simulink model "assignment2"  (R2020b)
settings: Solver=VariableStepAuto  StartTime=0.0  StopTime=10.0  RelTol=1e-3
undefined symbols (not defined in the file or in its folder): be, bv, Ie, Iv
settings Model: Creator=Sudhanshu  LastModifiedBy=Sudhanshu

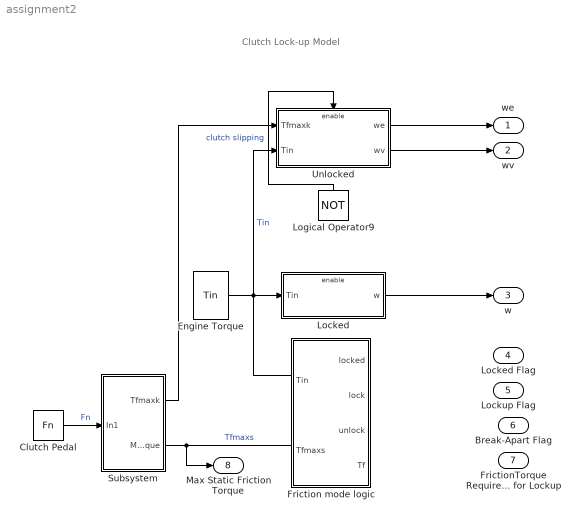
== system assignment2 ==
  note: Clutch Lock-up Model
  Clutch Pedal : FromWorkspace  VariableName=Fn  ZeroCross=off
  Engine Torque : FromWorkspace  VariableName=Tin  ZeroCross=off
  Friction mode logic : Subsystem
  Locked : Subsystem  TreatAsAtomicUnit=on
  Logical Operator9 : Logic  Operator=NOT  Inputs=1  IconShape=distinctive  OutDataTypeStr=boolean
  Subsystem : Subsystem
  Unlocked : Subsystem  TreatAsAtomicUnit=on
  we : Outport  InitialOutput=0  VectorParamsAs1DForOutWhenUnconnected=off
  wv : Outport  Port=2  InitialOutput=0  VectorParamsAs1DForOutWhenUnconnected=off
  w : Outport  Port=3  InitialOutput=0  VectorParamsAs1DForOutWhenUnconnected=off
  Locked Flag : Outport  Port=4  InitialOutput=0  VectorParamsAs1DForOutWhenUnconnected=off
  Lockup Flag : Outport  Port=5  InitialOutput=0  VectorParamsAs1DForOutWhenUnconnected=off
  Break-Apart Flag : Outport  Port=6  InitialOutput=0  VectorParamsAs1DForOutWhenUnconnected=off
  FrictionTorque Required for Lockup : Outport  Port=7  InitialOutput=0  VectorParamsAs1DForOutWhenUnconnected=off
  Max Static Friction Torque : Outport  Port=8  InitialOutput=0  VectorParamsAs1DForOutWhenUnconnected=off
  wires:
  Engine Torque/1 -> Locked/1(Tin), Unlocked/2(Tin)  "Tin"
  Unlocked/2(wv) -> wv/1
  Unlocked/1(we) -> we/1
  Logical Operator9/1 -> Unlocked/Enable  "clutch slipping"
  Locked/1(w) -> w/1
  Subsystem/1(Tfmaxk) -> Unlocked/1(Tfmaxk)
  Subsystem/2(Max Static Friction Torque) -> Max Static Friction Torque/1  "Tfmaxs"
  Clutch Pedal/1 -> Subsystem/1(In1)  "Fn"
  ? -> Locked/Enable, Logical Operator9/1, Locked Flag/1
  ? -> Lockup Flag/1
  ? -> Break-Apart Flag/1
  ? -> FrictionTorque Required for Lockup/1

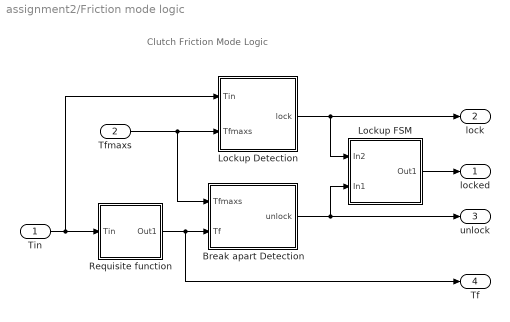
== system assignment2/Friction mode logic ==
  note: Clutch Friction Mode Logic
  Tin : Inport
  Tfmaxs : Inport  Port=2
  Break apart Detection : Subsystem
  Lockup Detection : Subsystem
  Lockup FSM : Subsystem
  Requisite function : Subsystem
  locked : Outport  InitialOutput=0  VectorParamsAs1DForOutWhenUnconnected=off
  lock : Outport  Port=2  InitialOutput=0  VectorParamsAs1DForOutWhenUnconnected=off
  unlock : Outport  Port=3  InitialOutput=0  VectorParamsAs1DForOutWhenUnconnected=off
  Tf : Outport  Port=4  InitialOutput=0  VectorParamsAs1DForOutWhenUnconnected=off
  wires:
  Break apart Detection/1(unlock) -> Lockup FSM/2(In1), unlock/1
  Tfmaxs/1 -> Break apart Detection/1(Tfmaxs), Lockup Detection/2(Tfmaxs)
  Lockup FSM/1(Out1) -> locked/1
  Lockup Detection/1(lock) -> Lockup FSM/1(In2), lock/1
  Requisite function/1(Out1) -> Break apart Detection/2(Tf), Tf/1
  Tin/1 -> Lockup Detection/1(Tin), Requisite function/1(Tin)

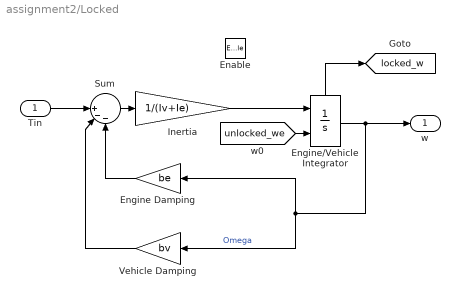
== system assignment2/Locked ==
  Tin : Inport
  Enable : EnablePort  StatesWhenEnabling=reset
  Engine Damping : Gain  Gain=be  SaturateOnIntegerOverflow=on  OutDataTypeStr=Inherit: Same as input  ParamDataTypeStr=Inherit: Same as input
  Engine/Vehicle Integrator : Integrator  InitialConditionSource=external  ShowStatePort=on
  Inertia : Gain  Gain=1/(Iv+Ie)  SaturateOnIntegerOverflow=on  OutDataTypeStr=Inherit: Same as input  ParamDataTypeStr=Inherit: Same as input
  Sum : Sum  Inputs=||+--  InputSameDT=on  SaturateOnIntegerOverflow=on  OutDataTypeStr=Inherit: Same as first input
  Vehicle Damping : Gain  Gain=bv  SaturateOnIntegerOverflow=on  OutDataTypeStr=Inherit: Same as input  ParamDataTypeStr=Inherit: Same as input
  w : Outport  InitialOutput=0  VectorParamsAs1DForOutWhenUnconnected=off
  tag scope: locked_w=global
  wires:
  Tin/1 -> Sum/1
  Engine/Vehicle Integrator/1 -> w/1, Engine Damping/1, Vehicle Damping/1  "Omega"
  Engine Damping/1 -> Sum/3
  Inertia/1 -> Engine/Vehicle Integrator/1
  Vehicle Damping/1 -> Sum/2
  Engine/Vehicle Integrator/State -> [locked_w]
  Sum/1 -> Inertia/1
  [unlocked_we] -> Engine/Vehicle Integrator/2

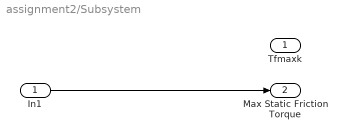
== system assignment2/Subsystem ==
  In1 : Inport
  Tfmaxk : Outport
  Max Static Friction Torque : Outport  Port=2
  wires:
  In1/1 -> Max Static Friction Torque/1

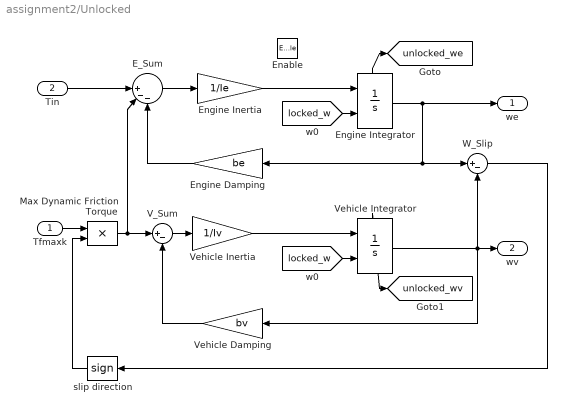
== system assignment2/Unlocked ==
  Tfmaxk : Inport
  Tin : Inport  Port=2
  Enable : EnablePort  StatesWhenEnabling=reset
  E_Sum : Sum  Inputs=||+--  InputSameDT=on  SaturateOnIntegerOverflow=on  OutDataTypeStr=Inherit: Same as first input
  Engine Damping : Gain  Gain=be  SaturateOnIntegerOverflow=on  OutDataTypeStr=Inherit: Same as input  ParamDataTypeStr=Inherit: Same as input
  Engine Inertia : Gain  Gain=1/Ie  SaturateOnIntegerOverflow=on  OutDataTypeStr=Inherit: Same as input  ParamDataTypeStr=Inherit: Same as input
  Engine Integrator : Integrator  InitialConditionSource=external  ShowStatePort=on
  Max Dynamic Friction Torque : Product  InputSameDT=on  RndMeth=Zero  SaturateOnIntegerOverflow=on  OutDataTypeStr=Inherit: Same as first input
  V_Sum : Sum  Inputs=|+-  InputSameDT=on  SaturateOnIntegerOverflow=on  OutDataTypeStr=Inherit: Same as first input
  Vehicle Damping : Gain  Gain=bv  SaturateOnIntegerOverflow=on  OutDataTypeStr=Inherit: Same as input  ParamDataTypeStr=Inherit: Same as input
  Vehicle Inertia : Gain  Gain=1/Iv  SaturateOnIntegerOverflow=on  OutDataTypeStr=Inherit: Same as input  ParamDataTypeStr=Inherit: Same as input
  Vehicle Integrator : Integrator  InitialConditionSource=external  ShowStatePort=on
  W_Slip : Sum  Inputs=|+-  InputSameDT=on  SaturateOnIntegerOverflow=on  OutDataTypeStr=Inherit: Same as first input
  slip direction : Signum
  we : Outport  InitialOutput=0  VectorParamsAs1DForOutWhenUnconnected=off
  wv : Outport  Port=2  InitialOutput=0  VectorParamsAs1DForOutWhenUnconnected=off
  tag scope: unlocked_we=global, unlocked_wv=global
  wires:
  V_Sum/1 -> Vehicle Inertia/1
  Engine Inertia/1 -> Engine Integrator/1
  [locked_w] -> Engine Integrator/2
  Engine Damping/1 -> E_Sum/3
  slip direction/1 -> Max Dynamic Friction Torque/2
  E_Sum/1 -> Engine Inertia/1
  Vehicle Integrator/State -> [unlocked_wv]
  [locked_w] -> Vehicle Integrator/2
  W_Slip/1 -> slip direction/1
  Tfmaxk/1 -> Max Dynamic Friction Torque/1
  Tin/1 -> E_Sum/1
  Vehicle Damping/1 -> V_Sum/2
  Vehicle Integrator/1 -> wv/1, W_Slip/2, Vehicle Damping/1
  Vehicle Inertia/1 -> Vehicle Integrator/1
  Engine Integrator/State -> [unlocked_we]
  Max Dynamic Friction Torque/1 -> V_Sum/1, E_Sum/2
  Engine Integrator/1 -> we/1, Engine Damping/1, W_Slip/1

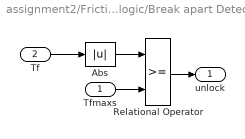
== system assignment2/Friction mode logic/Break apart Detection ==
  Tfmaxs : Inport
  Tf : Inport  Port=2
  Abs : Abs  SaturateOnIntegerOverflow=on
  Relational Operator : RelationalOperator  OutDataTypeStr=boolean  RndMeth=Nearest  InputSameDT=on
  unlock : Outport  InitialOutput=0  VectorParamsAs1DForOutWhenUnconnected=off
  wires:
  Abs/1 -> Relational Operator/1
  Tfmaxs/1 -> Relational Operator/2
  Tf/1 -> Abs/1
  Relational Operator/1 -> unlock/1

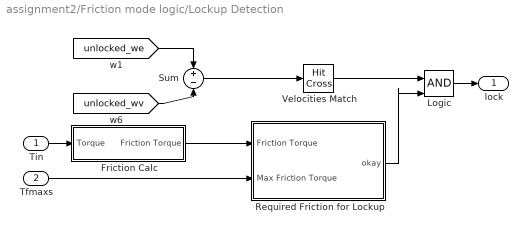
== system assignment2/Friction mode logic/Lockup Detection ==
  Tin : Inport
  Tfmaxs : Inport  Port=2
  Friction Calc : Subsystem
  Logic : Logic  IconShape=distinctive  OutDataTypeStr=boolean
  Required Friction for Lockup : Subsystem
  Sum : Sum  Inputs=+-  InputSameDT=on  SaturateOnIntegerOverflow=on  OutDataTypeStr=Inherit: Same as first input
  Velocities Match : HitCross
  lock : Outport  InitialOutput=0  VectorParamsAs1DForOutWhenUnconnected=off
  wires:
  Required Friction for Lockup/1(okay) -> Logic/2
  Sum/1 -> Velocities Match/1
  Velocities Match/1 -> Logic/1
  Tin/1 -> Friction Calc/1(Torque)
  [unlocked_we] -> Sum/1
  Logic/1 -> lock/1
  Tfmaxs/1 -> Required Friction for Lockup/2(Max Friction Torque)
  [unlocked_wv] -> Sum/2
  Friction Calc/1(Friction Torque) -> Required Friction for Lockup/1(Friction Torque)

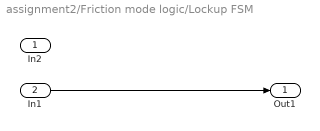
== system assignment2/Friction mode logic/Lockup FSM ==
  In2 : Inport
  In1 : Inport  Port=2
  Out1 : Outport
  wires:
  In1/1 -> Out1/1

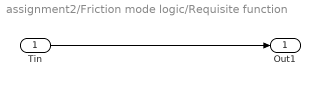
== system assignment2/Friction mode logic/Requisite function ==
  Tin : Inport
  Out1 : Outport
  wires:
  Tin/1 -> Out1/1

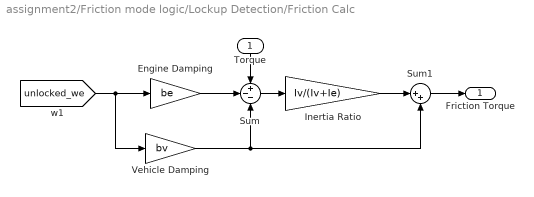
== system assignment2/Friction mode logic/Lockup Detection/Friction Calc ==
  Torque : Inport
  Engine Damping : Gain  Gain=be  SaturateOnIntegerOverflow=on  OutDataTypeStr=Inherit: Same as input  ParamDataTypeStr=Inherit: Same as input
  Inertia Ratio : Gain  Gain=Iv/(Iv+Ie)  SaturateOnIntegerOverflow=on  OutDataTypeStr=Inherit: Same as input  ParamDataTypeStr=Inherit: Same as input
  Sum : Sum  Inputs=+--  InputSameDT=on  SaturateOnIntegerOverflow=on  OutDataTypeStr=Inherit: Same as first input
  Sum1 : Sum  Inputs=|++  InputSameDT=on  SaturateOnIntegerOverflow=on  OutDataTypeStr=Inherit: Same as first input
  Vehicle Damping : Gain  Gain=bv  SaturateOnIntegerOverflow=on  OutDataTypeStr=Inherit: Same as input  ParamDataTypeStr=Inherit: Same as input
  Friction Torque : Outport  InitialOutput=0  VectorParamsAs1DForOutWhenUnconnected=off
  wires:
  [unlocked_we] -> Engine Damping/1, Vehicle Damping/1
  Vehicle Damping/1 -> Sum1/2, Sum/3
  Engine Damping/1 -> Sum/2
  Sum/1 -> Inertia Ratio/1
  Torque/1 -> Sum/1
  Inertia Ratio/1 -> Sum1/1
  Sum1/1 -> Friction Torque/1

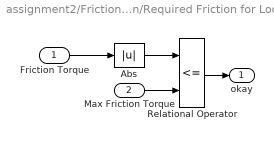
== system assignment2/Friction mode logic/Lockup Detection/Required Friction for Lockup ==
  Friction Torque : Inport
  Max Friction Torque : Inport  Port=2
  Abs : Abs  SaturateOnIntegerOverflow=on
  Relational Operator : RelationalOperator  Operator=<=  OutDataTypeStr=boolean  RndMeth=Nearest  InputSameDT=on
  okay : Outport  InitialOutput=0  VectorParamsAs1DForOutWhenUnconnected=off
  wires:
  Friction Torque/1 -> Abs/1
  Relational Operator/1 -> okay/1
  Abs/1 -> Relational Operator/1
  Max Friction Torque/1 -> Relational Operator/2
